simulink model "L0703"  (Simulink 10.2)
settings: Solver=VariableStepDiscrete  StartTime=0.0  StopTime=30  MaxStep=1  RelTol=1e-3
settings Model: Creator=Ranci  LastModifiedBy=Ranci
settings DataIOCC: SaveFormat=Dataset  SignalLoggingSaveFormat=Dataset  ReturnWorkspaceOutputs=on
settings OptimizationCC: LifeSpan=auto
settings DebuggingCC: UnderspecifiedInitializationDetection=Simplified  MergeDetectMultiDrivingBlocksExec=error  FcnCallInpInsideContextMsg=error  SFUnexpectedBacktrackingDiag=error  SFNoUnconditionalDefaultTransitionDiag=error  SFExecutionAtInitializationDiag=warning  ArithmeticOperatorsInVariantConditions=error
settings HardwareCC: ProdBitPerPointer=64  ProdBitPerSizeT=64  ProdBitPerPtrDiffT=64  ProdLargestAtomicFloat=Float  ProdIntDivRoundTo=Zero  ProdEndianess=LittleEndian  ProdWordSize=64  ProdHWDeviceType=Intel->x86-64 (Windows64)
settings ModelReferenceCC: PropagateSignalLabelsOutOfModel=on
settings SFSimCC: SimUseLocalCustomCode=on  CustomCodeUndefinedFunction=FilterOut
settings RTWCC: RTWUseLocalCustomCode=on
settings CodeAppCC: StateflowObjectComments=off
settings GRTTargetCC: TargetLangStandard=C99 (ISO)  CombineOutputUpdateFcns=on  GRTInterface=off
settings ConfigComp: CovMetricSettings=dwe  CovSaveCumulativeToWorkspaceVar=off  CovSaveSingleToWorkspaceVar=off  CovExternalEMLEnable=on

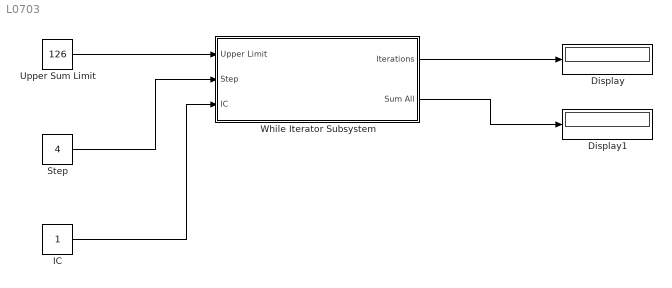
== system L0703 ==
  Display : Display
  Display1 : Display
  IC : Constant
  Step : Constant  Value=4
  Upper Sum Limit : Constant  Value=126
  While Iterator Subsystem : Subsystem  TreatAsAtomicUnit=on
  wires:
  Upper Sum Limit/1 -> While Iterator Subsystem/1(Upper Limit)
  Step/1 -> While Iterator Subsystem/2(Step)
  While Iterator Subsystem/1(Iterations) -> Display/1
  While Iterator Subsystem/2(Sum All) -> Display1/1
  IC/1 -> While Iterator Subsystem/3(IC)

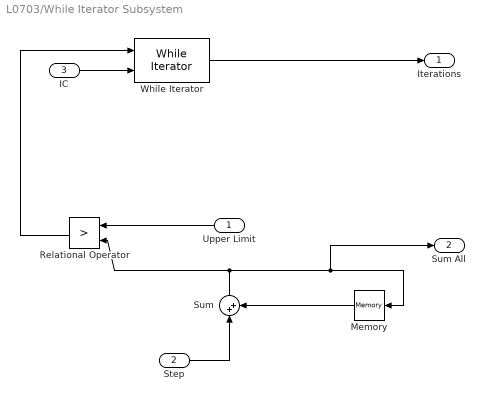
== system L0703/While Iterator Subsystem ==
  Upper Limit : Inport
  Step : Inport  Port=2
  IC : Inport  Port=3
  Memory : Memory  InheritSampleTime=on
  Relational Operator : RelationalOperator  Operator=>  OutDataTypeStr=boolean  RndMeth=Simplest
  Sum : Sum  Inputs=|++
  While Iterator : WhileIterator  MaxIters=-1  ResetStates=reset  ShowIterationPort=on
  Iterations : Outport
  Sum All : Outport  Port=2
  wires:
  Upper Limit/1 -> Relational Operator/1
  Sum/1 -> Sum All/1, Memory/1, Relational Operator/2
  Memory/1 -> Sum/2
  Step/1 -> Sum/1
  Relational Operator/1 -> While Iterator/1
  While Iterator/1 -> Iterations/1
  IC/1 -> While Iterator/2
